simulink library "Springs_Axle1_Linear"  (R2025b)
settings: Solver=VariableStepAuto  StartTime=0.0  StopTime=10.0  RelTol=1e-3
undefined symbols (not defined in the file): Spring
libraries: fl_lib x2, Spring_Linear x2
Description:
  | Component of Simscape Vehicle Templates Library
  | 
  | Copyright 2018-2025 The MathWorks, Inc.
settings Model: Creator=smiller  LastModifiedBy=smiller
settings SolverCC: AlgebraicLoopSolver=TrustRegion
settings DataIOCC: ReturnWorkspaceOutputs=off
settings OptimizationCC: ReuseModelBlockBuffer=off
settings DebuggingCC: UnconnectedInputMsg=warning  UnconnectedOutputMsg=warning  UnconnectedLineMsg=warning  ArithmeticOperatorsInVariantConditions=warning
settings ModelReferenceCC: EnableRefExpFcnMdlSchedulingChecks=on
settings SFSimCC: CustomCodeUndefinedFunction=UseInterfaceOnly
settings RTWCC: GPUComputeCapability=3.5  DLArmComputeVersion=19.05

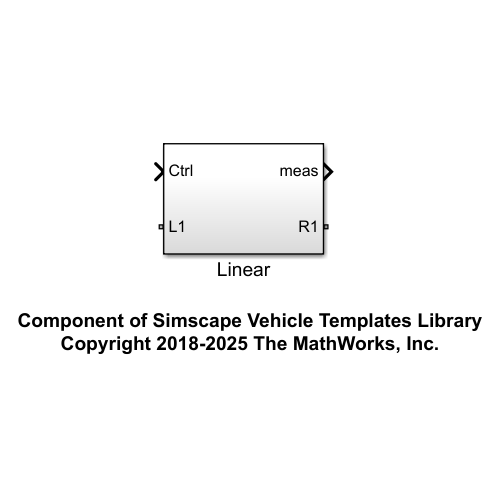
[thumbnail: Simulink's stored preview of the top-level diagram]
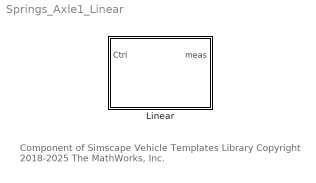
== system Springs_Axle1_Linear ==
  note: Component of Simscape Vehicle Templates Library
      | Copyright 2018-2025 The MathWorks, Inc.
  Linear : Subsystem  VariantControl=Linear

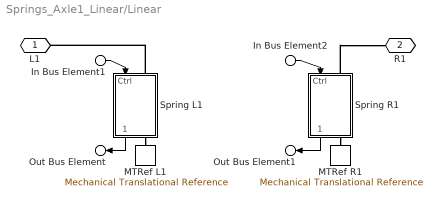
== system Springs_Axle1_Linear/Linear ==
  In Bus Element1 : Inport  PortName=Ctrl  Element=L1
  In Bus Element2 : Inport  PortName=Ctrl  Element=R1
  MTRef L1 : fl_lib/Mechanical/Translational Elements/Mechanical Translational Reference
  MTRef R1 : fl_lib/Mechanical/Translational Elements/Mechanical Translational Reference
  Spring L1 : Subsystem  mask{Spring=Spring.Front}
      mask prompts: Spring "Spring Parameters"
  Spring R1 : Subsystem  mask{Spring=Spring.Front}
      mask prompts: Spring "Spring Parameters"
  L1 : PMIOPort  Side=Left
  R1 : PMIOPort  Port=2  Side=Right
  Out Bus Element : Outport  VectorParamsAs1DForOutWhenUnconnected=off  PortName=meas  Element=L1
  Out Bus Element1 : Outport  VectorParamsAs1DForOutWhenUnconnected=off  PortName=meas  Element=R1
  wires:
  Spring R1/1(meas) -> Out Bus Element1/1
  In Bus Element2/1 -> Spring R1/1(Ctrl)
  Spring L1/1(meas) -> Out Bus Element/1
  In Bus Element1/1 -> Spring L1/1(Ctrl)
  connections:
  Spring L1/RConn1 -- MTRef L1/LConn1
  Spring L1/LConn1 -- L1/RConn1
  Spring R1/RConn1 -- MTRef R1/LConn1
  Spring R1/LConn1 -- R1/RConn1

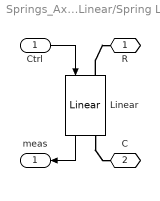
== system Springs_Axle1_Linear/Linear/Spring L1 ==
  Ctrl : Inport
  Linear : Spring_Linear/Linear  VariantControl=Linear  spr_def0=Spring.xPreload.Value  spr_frc0=Spring.fPreload.Value  spr_k=Spring.K.Value  spr_hp_top=Spring.sTop.Value  spr_hp_bot=Spring.sBottom.Value
  R : PMIOPort  Side=Left
  C : PMIOPort  Port=2  Side=Right
  meas : Outport  VectorParamsAs1DForOutWhenUnconnected=off
  wires:
  Ctrl/1 -> Linear/1
  Linear/1 -> meas/1
  connections:
  Linear/RConn1 -- C/RConn1
  Linear/LConn1 -- R/RConn1

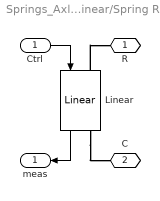
== system Springs_Axle1_Linear/Linear/Spring R1 ==
  Ctrl : Inport
  Linear : Spring_Linear/Linear  VariantControl=Linear  spr_def0=Spring.xPreload.Value  spr_frc0=Spring.fPreload.Value  spr_k=Spring.K.Value  spr_hp_top=Spring.sTop.Value  spr_hp_bot=Spring.sBottom.Value
  R : PMIOPort  Side=Left
  C : PMIOPort  Port=2  Side=Right
  meas : Outport  VectorParamsAs1DForOutWhenUnconnected=off
  wires:
  Linear/1 -> meas/1
  Ctrl/1 -> Linear/1
  connections:
  Linear/LConn1 -- R/RConn1
  Linear/RConn1 -- C/RConn1
